simulink model "gm_project_detect"  (R2020b)
settings: Solver=FixedStepDiscrete  StartTime=0.0  StopTime=SimTime  RelTol=1e-3
undefined symbols (not defined in the file or in its folder): CorrFilter, RxSignal, threshold, WindowLen
libraries: dspsrcs4 x2, dsphdlfiltering x1, simulink x1, hdlsllib x1
settings Model: Creator=cchung  LastModifiedBy=Aadhithan-PC
settings DataIOCC: SaveOutput=off  SaveTime=off
settings OptimizationCC: BlockReduction=off  ConditionallyExecuteInputs=off  DefaultParameterBehavior=Inlined
settings DebuggingCC: AlgebraicLoopMsg=error  InheritedTsInSrcMsg=none  SingleTaskRateTransMsg=error  PregeneratedLibrarySubsystemCodeDiagnostic=none  ArithmeticOperatorsInVariantConditions=warning
settings HardwareCC: ProdBitPerPointer=32  ProdBitPerSizeT=32  ProdBitPerPtrDiffT=32  ProdLargestAtomicFloat=None  ProdIntDivRoundTo=Undefined  ProdEndianess=Unspecified  ProdWordSize=32  ProdHWDeviceType=ASIC/FPGA->ASIC/FPGA  TargetBitPerPointer=64  TargetBitPerSizeT=64  TargetBitPerPtrDiffT=64  TargetLongLongMode=on  TargetIntDivRoundTo=Zero  TargetEndianess=LittleEndian  TargetWordSize=64  TargetHWDeviceType=Custom Processor->MATLAB Host Computer  ProdEqTarget=off
settings SFSimCC: SimUseLocalCustomCode=off  CustomCodeUndefinedFunction=UseInterfaceOnly
settings RTWCC: RTWUseLocalCustomCode=off

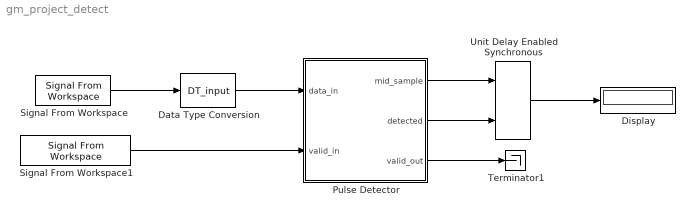
== system gm_project_detect ==
  Data Type Conversion : DataTypeConversion  OutDataTypeStr=DT_input  RndMeth=Nearest  SaturateOnIntegerOverflow=on
  Display : Display
  Pulse Detector : Subsystem
  Signal From Workspace : dspsrcs4/Signal From Workspace  X=RxSignal  Ts=1  nsamps=1  OutputAfterFinalValue=Setting to zero  ignoreOrWarnInputAndFrameLengths=off  OutputFrames=off
  Signal From Workspace1 : dspsrcs4/Signal From Workspace  X=true(size(RxSignal))  Ts=1  nsamps=1  OutputAfterFinalValue=Setting to zero  ignoreOrWarnInputAndFrameLengths=off  OutputFrames=off
  Terminator1 : Terminator
  Unit Delay Enabled Synchronous : hdlsllib/Discrete/Unit Delay Enabled Synchronous  InitialCondition=0.0  SampleTime=-1
      settings: SourceProductBaseCode=SL
  wires:
  Data Type Conversion/1 -> Pulse Detector/1(data_in)
  Pulse Detector/3(valid_out) -> Terminator1/1
  Signal From Workspace1/1 -> Pulse Detector/2(valid_in)
  Pulse Detector/2(detected) -> Unit Delay Enabled Synchronous/2
  Pulse Detector/1(mid_sample) -> Unit Delay Enabled Synchronous/1
  Signal From Workspace/1 -> Data Type Conversion/1
  Unit Delay Enabled Synchronous/1 -> Display/1

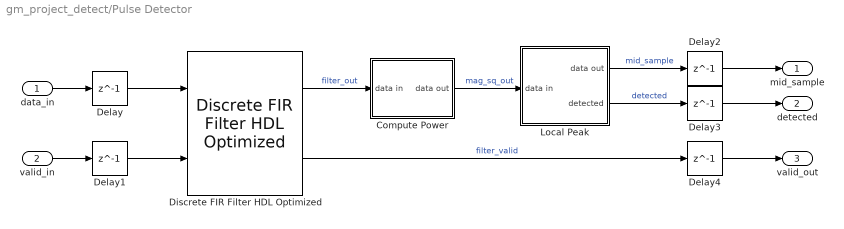
== system gm_project_detect/Pulse Detector ==
  data_in : Inport
  valid_in : Inport  Port=2
  Compute Power : Subsystem
  Delay{,1..4} (5 alike) : Delay  DelayLength=1
  Discrete FIR Filter HDL Optimized : dsphdlfiltering/Discrete FIR Filter HDL Optimized  NumeratorSource=Property  Numerator=CorrFilter  NumeratorPrototype=[]  FilterStructure=Direct form systolic  SerializationOption=Minimum number of cycles between valid input samples  NumberOfCycles=2  NumberOfMultipliers=2  SimulateUsing=Code generation  roundingMode=Floor  overflowMode=off  CoefficientsDataTypeStr=DT_coeff  CoefficientsMin=[]  CoefficientsMax=[]  OutputMin=[]  OutputMax=[]  ResetInputPort=off  HDLGlobalReset=off
      settings: SourceProductBaseCode=DS
  Local Peak : Subsystem
  mid_sample : Outport
  detected : Outport  Port=2
  valid_out : Outport  Port=3
  wires:
  Delay4/1 -> valid_out/1
  Delay3/1 -> detected/1
  Delay2/1 -> mid_sample/1
  Delay1/1 -> Discrete FIR Filter HDL Optimized/2
  Delay/1 -> Discrete FIR Filter HDL Optimized/1
  Discrete FIR Filter HDL Optimized/2 -> Delay4/1  "filter_valid"
  valid_in/1 -> Delay1/1
  data_in/1 -> Delay/1
  Local Peak/1(data out) -> Delay2/1  "mid_sample"
  Compute Power/1(data out) -> Local Peak/1(data in)  "mag_sq_out"
  Discrete FIR Filter HDL Optimized/1 -> Compute Power/1(data in)  "filter_out"
  Local Peak/2(detected) -> Delay3/1  "detected"

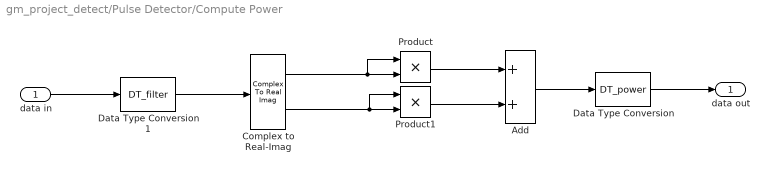
== system gm_project_detect/Pulse Detector/Compute Power ==
  data in : Inport
  Add : Sum
  Complex to Real-Imag : ComplexToRealImag
  Data Type Conversion : DataTypeConversion  OutDataTypeStr=DT_power
  Data Type Conversion1 : DataTypeConversion  OutDataTypeStr=DT_filter
  Product : Product
  Product1 : Product
  data out : Outport  VectorParamsAs1DForOutWhenUnconnected=off
  wires:
  Data Type Conversion/1 -> data out/1
  Data Type Conversion1/1 -> Complex to Real-Imag/1
  data in/1 -> Data Type Conversion1/1
  Add/1 -> Data Type Conversion/1
  Product/1 -> Add/1
  Product1/1 -> Add/2
  Complex to Real-Imag/2 -> Product1/2, Product1/1
  Complex to Real-Imag/1 -> Product/2, Product/1

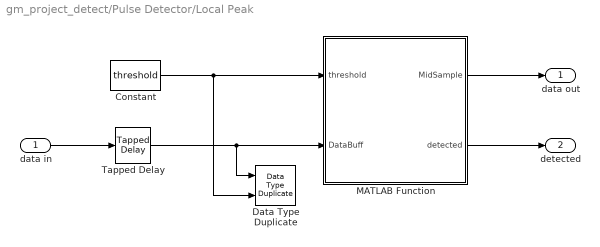
== system gm_project_detect/Pulse Detector/Local Peak ==
  data in : Inport
  Constant : Constant  Value=threshold  OutDataTypeStr=Inherit: Inherit via back propagation  SampleTime=-1
  Data Type Duplicate : DataTypeDuplicate
  MATLAB Function : MATLAB Function  TreatAsAtomicUnit=on
  Tapped Delay : simulink/Discrete/Tapped Delay  vinit=0.0  samptime=-1  NumDelays=WindowLen  DelayOrder=Oldest  includeCurrent=off
  data out : Outport  VectorParamsAs1DForOutWhenUnconnected=off
  detected : Outport  Port=2  VectorParamsAs1DForOutWhenUnconnected=off
  wires:
  MATLAB Function/2(detected) -> detected/1
  MATLAB Function/1(MidSample) -> data out/1
  Constant/1 -> MATLAB Function/1(threshold), Data Type Duplicate/2
  Tapped Delay/1 -> MATLAB Function/2(DataBuff), Data Type Duplicate/1
  data in/1 -> Tapped Delay/1

== matlab function gm_project_detect/Pulse Detector/Local Peak/MATLAB Function ==
  settings: fimath=fimath('RoundingMethod', 'Floor','OverflowAction', 'Wrap','ProductMode', 'FullPrecision', 'SumMode', 'FullPrecision')
  data: threshold input; DataBuff input; WindowLen parameter; MidSample output; detected output

% Hardware friendly implementation of peak finder
%
% Function inputs:
% * WindowLen - non-tunable parameter defined under Simulink->Edit Data
% * threhold  - input port (connected to constant)
% * DataBuff  - input port (buffering done using Simulink block)
%
% Function outputs:
% * "detected" is set when MidSample is local max

function [MidSample,detected] = fcn(threshold, DataBuff, WindowLen)
%#codegen


MidIdx = ceil(WindowLen/2);

% Compare each value in the window to the middle sample via subtraction
MidSample = DataBuff(MidIdx);
CompareOut = DataBuff - MidSample; % this is a vector

% if all values in the result are negative and the middle sample is
% greater than a threshold, it is a local max
if all(CompareOut <= 0) && (MidSample > threshold)
    detected = true;
else
    detected = false;
end
